simulink subsystem "Encoder"  (R2024b)
settings: Solver=VariableStepAuto  StartTime=0.0  StopTime=10.0  RelTol=1e-3
values from neighbouring files (symbols this model uses):
  Ts = Ts_values(i)    [A_final_results.m]
settings Model: Creator=Riccardo Grosso  LastModifiedBy=Riccardo Grosso

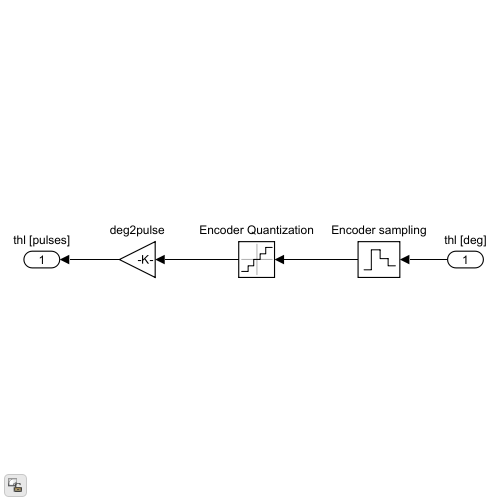
[thumbnail: Simulink's stored preview of the top-level diagram]
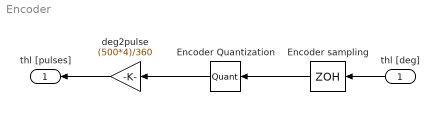
== system Encoder ==
  thl [deg] : Inport
  Encoder Quantization : Quantizer  QuantizationInterval=360/(500*4)
  Encoder sampling : ZeroOrderHold  SampleTime=Ts
  deg2pulse : Gain  Gain=(500*4)/360
  thl [pulses] : Outport
  wires:
  Encoder sampling/1 -> Encoder Quantization/1
  Encoder Quantization/1 -> deg2pulse/1
  thl [deg]/1 -> Encoder sampling/1
  deg2pulse/1 -> thl [pulses]/1
